simulink model "TADPOLEValveControl"  (R2024b)
settings: Solver=VariableStepAuto  StartTime=0.0  StopTime=100  RelTol=1e-3
values from neighbouring files (symbols this model uses):
  actuator_delay = 0.1131    [TADPOLEControl.m]
  ipaDensityArray = 0.02836    [ipaangle2mdot.m]
  ipaPressureArray = 0.638    [ipaangle2mdot.m]
  oxDensityArray = fuelData(1,:)    [MDotODE.m]    (also in oxangle2mdot.m)
  oxPressureArray = fuelData(2,:)    [MDotODE.m]    (also in oxangle2mdot.m)
undefined symbols (not defined in the file or in its folder): consts, DiscIntNeverNeededParam, Ki1, KiIPA, KiOX, Kp1, KpIPA, KpOX, model_error, simData, thrustArray
libraries: dspobslib x5, dspsrcs4 x2
settings Model: Creator=pplat  LastModifiedBy=pplat
settings DebuggingCC: AlgebraicLoopMsg=none

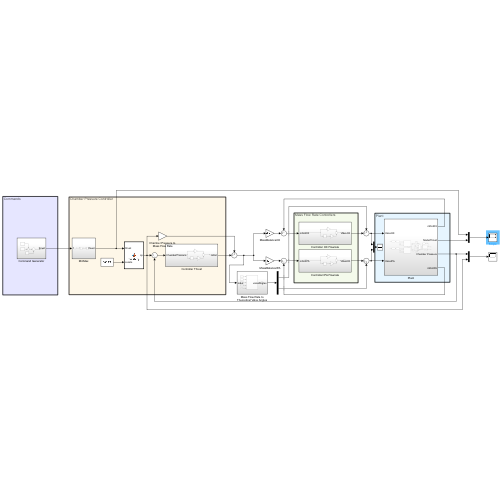
[thumbnail: Simulink's stored preview of the top-level diagram]
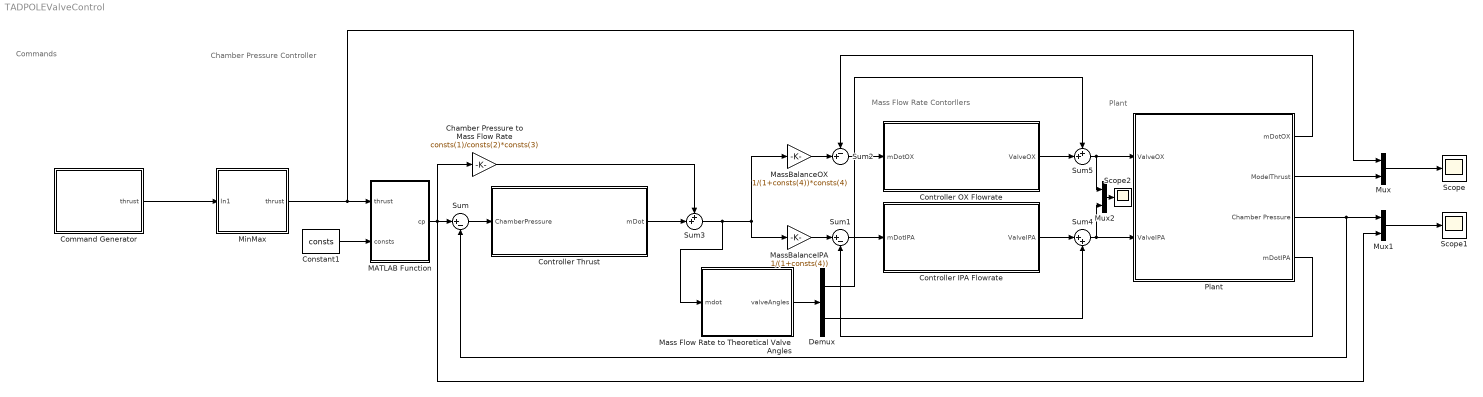
== system TADPOLEValveControl ==
  note: Plant
  note: Mass Flow Rate Contorllers
  note: Chamber Pressure Controller
  note: Commands
  Chamber Pressure to Mass Flow Rate : Gain  Gain=consts(1)/consts(2)*consts(3)
  Command Generator : Subsystem
  Constant1 : Constant  Value=consts
  Controller IPA Flowrate : Subsystem
  Controller OX Flowrate : Subsystem
  Controller Thrust : Subsystem
  Demux : Demux  Outputs=2
  MATLAB Function : MATLAB Function  TreatAsAtomicUnit=on
  "Mass Flow Rate to Theoretical Valve Angles " : Subsystem
  MassBalanceIPA : Gain  Gain=1/(1+consts(4))
  MassBalanceOX : Gain  Gain=1/(1+consts(4))*consts(4)
  MinMax : Subsystem
  Mux : Mux  Inputs=2
  Mux1 : Mux  Inputs=2
  Mux2 : Mux  Inputs=2
  Plant : Subsystem
  Scope : Scope
  Scope1 : Scope
  Scope2 : Scope
  Sum : Sum  Inputs=|+-
  Sum1 : Sum  Inputs=|+-
  Sum2 : Sum  Inputs=-+|
  Sum3 : Sum  Inputs=++|
  Sum4 : Sum  Inputs=|++
  Sum5 : Sum  Inputs=++|
  wires:
  Constant1/1 -> MATLAB Function/2(consts)
  Command Generator/1(thrust) -> MinMax/1(In1)
  Plant/2(ModelThrust) -> Mux/2
  MinMax/1(thrust) -> MATLAB Function/1(thrust), Mux/1
  Mux/1 -> Scope/1
  Sum/1 -> Controller Thrust/1(ChamberPressure)
  Sum1/1 -> Controller IPA Flowrate/1(mDotIPA)
  MassBalanceOX/1 -> Sum2/2
  Sum2/1 -> Controller OX Flowrate/1(mDotOX)
  Plant/1(mDotOX) -> Sum2/1
  Plant/4(mDotIPA) -> Sum1/2
  Plant/3(Chamber Pressure) -> Sum/2, Mux1/1
  Mux1/1 -> Scope1/1
  MATLAB Function/1(cp) -> Chamber Pressure to Mass Flow Rate/1, Mux1/2, Sum/1
  Controller Thrust/1(mDot) -> Sum3/2
  Chamber Pressure to Mass Flow Rate/1 -> Sum3/1
  Sum3/1 -> "Mass Flow Rate to Theoretical Valve Angles "/1(mdot), MassBalanceIPA/1, MassBalanceOX/1
  MassBalanceIPA/1 -> Sum1/1
  Controller IPA Flowrate/1(ValveIPA) -> Sum4/1
  Sum4/1 -> Mux2/2, Plant/2(ValveIPA)
  Controller OX Flowrate/1(ValveOX) -> Sum5/2
  Sum5/1 -> Mux2/1, Plant/1(ValveOX)
  "Mass Flow Rate to Theoretical Valve Angles "/1(valveAngles) -> Demux/1
  Demux/1 -> Sum5/1
  Demux/2 -> Sum4/2
  Mux2/1 -> Scope2/1

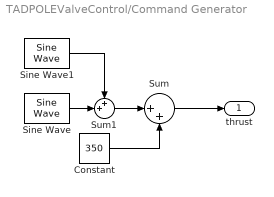
== system TADPOLEValveControl/Command Generator ==
  Constant : Constant  Value=350
  Sine Wave : dspsrcs4/Sine Wave  Amplitude=75  Frequency=0.05  Phase=0  SampleMode=Discrete  OutComplex=Real  CompMethod=Trigonometric fcn  TableSize=Speed  SampleTime=1/60  SamplesPerFrame=1  ResetState=Restart at time zero  OutputFrames=off  dataType=double  wordLen=16  udDataType=sfix(16)  fracBitsMode=Best precision  numFracBits=15  OutDataTypeStr=double  LastOutDataTypeStr=double
  Sine Wave1 : dspsrcs4/Sine Wave  Amplitude=40  Frequency=0.21  Phase=0  SampleMode=Discrete  OutComplex=Real  CompMethod=Trigonometric fcn  TableSize=Speed  SampleTime=1/60  SamplesPerFrame=1  ResetState=Restart at time zero  OutputFrames=off  dataType=double  wordLen=16  udDataType=sfix(16)  fracBitsMode=Best precision  numFracBits=15  OutDataTypeStr=double  LastOutDataTypeStr=double
  Sum : Sum  Inputs=|++
  Sum1 : Sum  Inputs=++|
  thrust : Outport
  wires:
  Sum/1 -> thrust/1
  Constant/1 -> Sum/2
  Sine Wave/1 -> Sum1/2
  Sum1/1 -> Sum/1
  Sine Wave1/1 -> Sum1/1

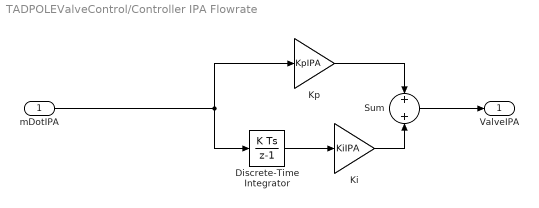
== system TADPOLEValveControl/Controller IPA Flowrate ==
  mDotIPA : Inport
  Discrete-Time Integrator : DiscreteIntegrator  SampleTime=-1  ICPrevOutput=DiscIntNeverNeededParam  ICPrevScaledInput=DiscIntNeverNeededParam
  Ki : Gain  Gain=KiIPA
  Kp : Gain  Gain=KpIPA
  Sum : Sum  Inputs=+|+
  ValveIPA : Outport
  wires:
  mDotIPA/1 -> Discrete-Time Integrator/1, Kp/1
  Kp/1 -> Sum/1
  Ki/1 -> Sum/2
  Sum/1 -> ValveIPA/1
  Discrete-Time Integrator/1 -> Ki/1

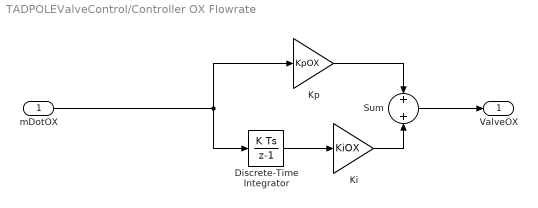
== system TADPOLEValveControl/Controller OX Flowrate ==
  mDotOX : Inport
  Discrete-Time Integrator : DiscreteIntegrator  SampleTime=-1  ICPrevOutput=DiscIntNeverNeededParam  ICPrevScaledInput=DiscIntNeverNeededParam
  Ki : Gain  Gain=KiOX
  Kp : Gain  Gain=KpOX
  Sum : Sum  Inputs=+|+
  ValveOX : Outport
  wires:
  mDotOX/1 -> Discrete-Time Integrator/1, Kp/1
  Kp/1 -> Sum/1
  Ki/1 -> Sum/2
  Sum/1 -> ValveOX/1
  Discrete-Time Integrator/1 -> Ki/1

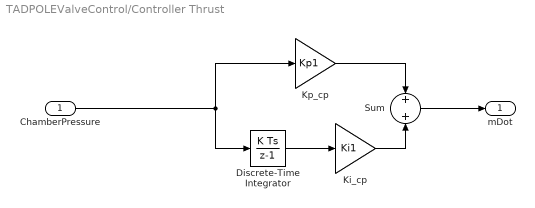
== system TADPOLEValveControl/Controller Thrust ==
  ChamberPressure : Inport
  Discrete-Time Integrator : DiscreteIntegrator  SampleTime=-1  ICPrevOutput=DiscIntNeverNeededParam  ICPrevScaledInput=DiscIntNeverNeededParam
  Ki_cp : Gain  Gain=Ki1
  Kp_cp : Gain  Gain=Kp1
  Sum : Sum  Inputs=+|+
  mDot : Outport
  wires:
  ChamberPressure/1 -> Discrete-Time Integrator/1, Kp_cp/1
  Kp_cp/1 -> Sum/1
  Ki_cp/1 -> Sum/2
  Sum/1 -> mDot/1
  Discrete-Time Integrator/1 -> Ki_cp/1

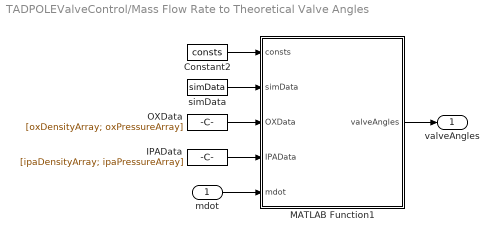
== system TADPOLEValveControl/Mass Flow Rate to Theoretical Valve Angles  ==
  mdot : Inport
  Constant2 : Constant  Value=consts
  IPAData : Constant  Value=[ipaDensityArray; ipaPressureArray]
  MATLAB Function1 : MATLAB Function  TreatAsAtomicUnit=on
  OXData : Constant  Value=[oxDensityArray; oxPressureArray]
  simData : Constant  Value=simData
  valveAngles : Outport
  wires:
  Constant2/1 -> MATLAB Function1/1(consts)
  simData/1 -> MATLAB Function1/2(simData)
  IPAData/1 -> MATLAB Function1/4(IPAData)
  OXData/1 -> MATLAB Function1/3(OXData)
  mdot/1 -> MATLAB Function1/5(mdot)
  MATLAB Function1/1(valveAngles) -> valveAngles/1

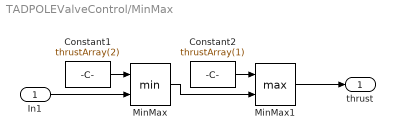
== system TADPOLEValveControl/MinMax ==
  In1 : Inport
  Constant1 : Constant  Value=thrustArray(2)
  Constant2 : Constant  Value=thrustArray(1)
  MinMax : MinMax  Inputs=2
  MinMax1 : MinMax  Function=max  Inputs=2
  thrust : Outport
  wires:
  Constant2/1 -> MinMax1/1
  Constant1/1 -> MinMax/1
  MinMax/1 -> MinMax1/2
  In1/1 -> MinMax/2
  MinMax1/1 -> thrust/1

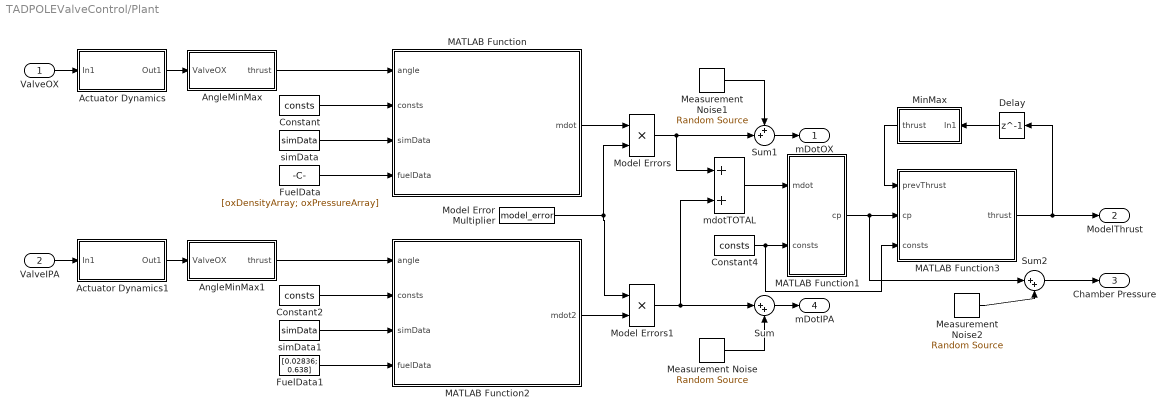
== system TADPOLEValveControl/Plant ==
  ValveOX : Inport
  ValveIPA : Inport  Port=2
  Actuator Dynamics : Subsystem
  Actuator Dynamics1 : Subsystem
  AngleMinMax : Subsystem
  AngleMinMax1 : Subsystem
  Constant : Constant  Value=consts
  Constant2 : Constant  Value=consts
  Constant4 : Constant  Value=consts
  Delay : Delay  DelayLength=1  InitialCondition=0  InputProcessing=Columns as channels (frame based)
  FuelData : Constant  Value=[oxDensityArray; oxPressureArray]
  FuelData1 : Constant  Value=[0.02836; 0.638]
  MATLAB Function : MATLAB Function  TreatAsAtomicUnit=on
  MATLAB Function1 : MATLAB Function  TreatAsAtomicUnit=on
  MATLAB Function2 : MATLAB Function  TreatAsAtomicUnit=on
  MATLAB Function3 : MATLAB Function  TreatAsAtomicUnit=on
  Measurement Noise : dspobslib/Random Source  SrcType=Gaussian  NormMethod=Ziggurat  CltLength=12  MinVal=0  MaxVal=1  MeanVal=0  VarVal=noise_var_outputs  RepMode=Not repeatable  rawSeed=1  IsInherit=off  SampMode=Continuous  SampTime=1  SampFrame=1  DataType=Double  OutComplex=Real  OutputFrames=off
  Measurement Noise1 : dspobslib/Random Source  SrcType=Gaussian  NormMethod=Ziggurat  CltLength=12  MinVal=0  MaxVal=1  MeanVal=0  VarVal=noise_var_outputs  RepMode=Not repeatable  rawSeed=1  IsInherit=off  SampMode=Continuous  SampTime=1  SampFrame=1  DataType=Double  OutComplex=Real  OutputFrames=off
  Measurement Noise2 : dspobslib/Random Source  SrcType=Gaussian  NormMethod=Ziggurat  CltLength=12  MinVal=0  MaxVal=1  MeanVal=0  VarVal=noise_var_outputs  RepMode=Not repeatable  rawSeed=1  IsInherit=off  SampMode=Continuous  SampTime=1  SampFrame=1  DataType=Double  OutComplex=Real  OutputFrames=off
  MinMax : Subsystem
  Model Error Multiplier : Constant  Value=model_error
  Model Errors : Product
  Model Errors1 : Product
  Sum : Sum  Inputs=|++
  Sum1 : Sum  Inputs=++|
  Sum2 : Sum  Inputs=|++
  mdotTOTAL : Sum
  simData : Constant  Value=simData
  simData1 : Constant  Value=simData
  mDotOX : Outport
  ModelThrust : Outport  Port=2
  Chamber Pressure : Outport  Port=3
  mDotIPA : Outport  Port=4
  wires:
  Constant/1 -> MATLAB Function/2(consts)
  FuelData/1 -> MATLAB Function/4(fuelData)
  FuelData1/1 -> MATLAB Function2/4(fuelData)
  Constant2/1 -> MATLAB Function2/2(consts)
  Constant4/1 -> MATLAB Function3/3(consts), MATLAB Function1/2(consts)
  mdotTOTAL/1 -> MATLAB Function1/1(mdot)
  Delay/1 -> MinMax/1(In1)
  MinMax/1(thrust) -> MATLAB Function3/1(prevThrust)
  simData/1 -> MATLAB Function/3(simData)
  simData1/1 -> MATLAB Function2/3(simData)
  MATLAB Function3/1(thrust) -> ModelThrust/1, Delay/1
  MATLAB Function1/1(cp) -> Sum2/1, MATLAB Function3/2(cp)
  ValveOX/1 -> Actuator Dynamics/1(In1)
  Actuator Dynamics/1(Out1) -> AngleMinMax/1(ValveOX)
  ValveIPA/1 -> Actuator Dynamics1/1(In1)
  Actuator Dynamics1/1(Out1) -> AngleMinMax1/1(ValveOX)
  Sum/1 -> mDotIPA/1
  Measurement Noise/1 -> Sum/2
  Sum1/1 -> mDotOX/1
  Measurement Noise1/1 -> Sum1/1
  Measurement Noise2/1 -> Sum2/2
  Sum2/1 -> Chamber Pressure/1
  Model Errors/1 -> Sum1/2, mdotTOTAL/1
  MATLAB Function/1(mdot) -> Model Errors/1
  MATLAB Function2/1(mdot2) -> Model Errors1/2
  Model Errors1/1 -> mdotTOTAL/2, Sum/1
  Model Error Multiplier/1 -> Model Errors1/1, Model Errors/2
  AngleMinMax/1(thrust) -> MATLAB Function/1(angle)
  AngleMinMax1/1(thrust) -> MATLAB Function2/1(angle)

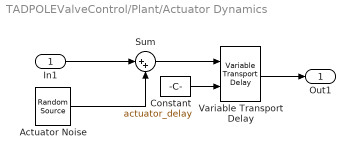
== system TADPOLEValveControl/Plant/Actuator Dynamics ==
  In1 : Inport
  Actuator Noise : dspobslib/Random Source  SrcType=Gaussian  NormMethod=Ziggurat  CltLength=12  MinVal=0  MaxVal=1  MeanVal=0  VarVal=noise_var_actuators  RepMode=Not repeatable  rawSeed=1  IsInherit=off  SampMode=Continuous  SampTime=1  SampFrame=1  DataType=Double  OutComplex=Real  OutputFrames=off
  Constant : Constant  Value=actuator_delay
  Sum : Sum  Inputs=|++
  Variable Transport Delay : VariableTransportDelay  VariableDelayType=Variable transport delay  MaximumDelay=10  MaximumPoints=2048
  Out1 : Outport
  wires:
  Actuator Noise/1 -> Sum/2
  In1/1 -> Sum/1
  Constant/1 -> Variable Transport Delay/2
  Variable Transport Delay/1 -> Out1/1
  Sum/1 -> Variable Transport Delay/1

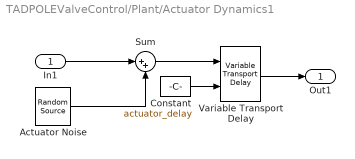
== system TADPOLEValveControl/Plant/Actuator Dynamics1 ==
  In1 : Inport
  Actuator Noise : dspobslib/Random Source  SrcType=Gaussian  NormMethod=Ziggurat  CltLength=12  MinVal=0  MaxVal=1  MeanVal=0  VarVal=noise_var_actuators  RepMode=Not repeatable  rawSeed=1  IsInherit=off  SampMode=Continuous  SampTime=1  SampFrame=1  DataType=Double  OutComplex=Real  OutputFrames=off
  Constant : Constant  Value=actuator_delay
  Sum : Sum  Inputs=|++
  Variable Transport Delay : VariableTransportDelay  VariableDelayType=Variable transport delay  MaximumDelay=10  MaximumPoints=2048
  Out1 : Outport
  wires:
  Actuator Noise/1 -> Sum/2
  In1/1 -> Sum/1
  Constant/1 -> Variable Transport Delay/2
  Variable Transport Delay/1 -> Out1/1
  Sum/1 -> Variable Transport Delay/1

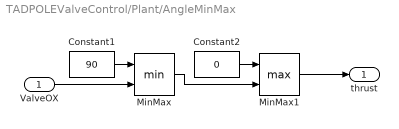
== system TADPOLEValveControl/Plant/AngleMinMax ==
  ValveOX : Inport
  Constant1 : Constant  Value=90
  Constant2 : Constant  Value=0
  MinMax : MinMax  Inputs=2
  MinMax1 : MinMax  Function=max  Inputs=2
  thrust : Outport
  wires:
  Constant2/1 -> MinMax1/1
  Constant1/1 -> MinMax/1
  MinMax/1 -> MinMax1/2
  ValveOX/1 -> MinMax/2
  MinMax1/1 -> thrust/1

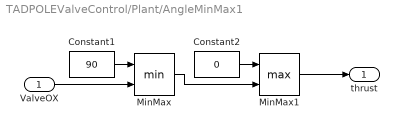
== system TADPOLEValveControl/Plant/AngleMinMax1 ==
  ValveOX : Inport
  Constant1 : Constant  Value=90
  Constant2 : Constant  Value=0
  MinMax : MinMax  Inputs=2
  MinMax1 : MinMax  Function=max  Inputs=2
  thrust : Outport
  wires:
  Constant2/1 -> MinMax1/1
  Constant1/1 -> MinMax/1
  MinMax/1 -> MinMax1/2
  ValveOX/1 -> MinMax/2
  MinMax1/1 -> thrust/1

== system TADPOLEValveControl/Plant/MinMax ==
  In1 : Inport
  Constant1 : Constant  Value=thrustArray(2)
  Constant2 : Constant  Value=thrustArray(1)
  MinMax : MinMax  Inputs=2
  MinMax1 : MinMax  Function=max  Inputs=2
  thrust : Outport
  wires:
  Constant2/1 -> MinMax1/1
  Constant1/1 -> MinMax/1
  MinMax/1 -> MinMax1/2
  In1/1 -> MinMax/2
  MinMax1/1 -> thrust/1

== matlab function TADPOLEValveControl/Plant/MATLAB Function ==
  data: angle input; mdot output; consts input; simData input; fuelData input
function mdot = oxangle2mdot(angle, consts, simData, fuelData)

    % Conversion Factors and LookUp Arrays
    conversionFactors = [0.004329 60 0.000453592 61023.7];
    subCritVArray = [0.000, 0.070, 0.161, 0.378, 0.670, 1.000, 1.450, 2.050, 2.780, 3.710, 4.960];
    valveAngleArray = [0, 9, 18, 27, 36, 45, 54, 63, 72, 81, 90];
    tempArray = [55, 60, 65, 70, 75, 80, 85, 90, 95, 100, 105, 110, ...
    115, 120, 125, 130, 135, 140, 145, 150];
    oxDensityArray = fuelData(1,:);
    oxPressureArray = fuelData(2,:);

    % cV lookup based off of angle
    subCritV = interp1(valveAngleArray, subCritVArray, angle);

    % ox
    throat = 0.00989;
    cd = 0.975;

    % density and vapour pressure ox
    simData(4);
    density_cv = interp1(tempArray, oxDensityArray, simData(4));
    p_vap = interp1(tempArray, oxPressureArray, simData(4));
    density_valve = interp1(tempArray, oxDensityArray, simData(3));

    %Generates mdot
    alpha = conversionFactors(1)*conversionFactors(2);
    gamma = cd^2*throat^2*2*density_cv*(consts(3)*12);
    beta = conversionFactors(3)*conversionFactors(4);
    deltaP = simData(1)-p_vap;
    mdot = sqrt(subCritV^2*density_valve*(deltaP)*gamma /...
        (alpha^2*gamma*beta + subCritV^2*density_valve));
end

== matlab function TADPOLEValveControl/MATLAB Function ==
  data: thrust input; cp output; consts input
function cp = thrust2cp(thrust, consts)
  
    thrustArray = [220, 550];
    c_fArray = [1.12, 1.3];
    c_f = interp1(thrustArray, c_fArray, thrust);
    cp = thrust / (c_f*consts(1));
end

== matlab function TADPOLEValveControl/Plant/MATLAB Function1 ==
  data: mdot input; cp output; consts input
function cp = mdot2cp(mdot, consts)
    
    cp = mdot*consts(2) / (consts(1)*consts(3));
end

== matlab function TADPOLEValveControl/Plant/MATLAB Function2 ==
  data: angle input; mdot2 output; consts input; simData input; fuelData input
function mdot2 = ipaangle2mdot(angle, consts, simData, fuelData)

    % Conversion Factors and LookUp Arrays
    conversionFactors = [0.004329 60 0.000453592 61023.7];
    subCritVArray = [0.000, 0.070, 0.161, 0.378, 0.670, 1.000, 1.450, 2.050, 2.780, 3.710, 4.960];
    valveAngleArray = [0, 9, 18, 27, 36, 45, 54, 63, 72, 81, 90];
    tempArray = [55, 60, 65, 70, 75, 80, 85, 90, 95, 100, 105, 110, ...
    115, 120, 125, 130, 135, 140, 145, 150];
    ipaDensityArray = fuelData(1,:);
    ipaPressureArray = fuelData(2,:);

    % cV lookup based off of angle
    subCritV = interp1(valveAngleArray, subCritVArray, angle);

    % ox
    throat = 0.00989;
    cd = 0.975;

    % density and vapour pressure ox
    simData(4);
    density_cv = ipaDensityArray;
    p_vap = ipaPressureArray;
    density_valve = ipaDensityArray;

    %Generates mdot
    alpha = conversionFactors(1)*conversionFactors(2);
    gamma = cd^2*throat^2*2*density_cv*(consts(3)*12);
    beta = conversionFactors(3)*conversionFactors(4);
    deltaP = simData(1)-p_vap;
    mdot2 = sqrt(subCritV^2*density_valve*(deltaP)*gamma /...
        (alpha^2*gamma*beta + subCritV^2*density_valve));
end

== matlab function TADPOLEValveControl/Plant/MATLAB Function3 ==
  data: prevThrust input; cp input; thrust output; consts input
function thrust = cp2thrust(prevThrust, cp, consts)
  
    thrustArray = [220, 550];
    c_fArray = [1.12, 1.3];
    c_f = interp1(thrustArray, c_fArray, prevThrust);
    thrust = cp*c_f*consts(1);
end

== matlab function TADPOLEValveControl/Mass Flow Rate to Theoretical Valve Angles /MATLAB Function1 ==
  data: consts input; simData input; OXData input; IPAData input; mdot input; valveAngles output
function valveAngles = mdot2valves(consts, simData, OXData, IPAData, mdot)
   
    % Conversion Factors and LookUp Arrays
    conversionFactors = [0.004329 60 0.000453592 61023.7];
    subCritVArray = [0.000, 0.070, 0.161, 0.378, 0.670, 1.000, 1.450, 2.050, 2.780, 3.710, 4.960];
    valveAngleArray = [0, 9, 18, 27, 36, 45, 54, 63, 72, 81, 90];
    tempArray = [55, 60, 65, 70, 75, 80, 85, 90, 95, 100, 105, 110, ...
    115, 120, 125, 130, 135, 140, 145, 150];
    oxDensityArray = OXData(1,:);
    oxPressureArray = OXData(2,:);

    % Mass balance
    mdot_OX = mdot / (1+consts(4))*consts(4);
    mdot_IPA = mdot / (1+consts(4));

    % ox/ipa 
    throat = 0.00989;
    cd = 0.975;
    densityOX_cv = interp1(tempArray, oxDensityArray, simData(4));
    densityIPA_cv = IPAData(1);
    densityOX_valve = interp1(tempArray, oxDensityArray, simData(3));
    densityIPA_valve = IPAData(1);
    P_vap_OX = interp1(tempArray, oxPressureArray, simData(4));
    P_vap_IPA = IPAData(2);

    % Cavitating venturis
    P_in_OX = (mdot_OX / (cd*throat))^2 / (2*densityOX_cv*(consts(3)*12))...
        + P_vap_OX;
    P_in_IPA = (mdot_IPA / (cd*throat))^2 / (2*densityIPA_cv*(consts(3)*12))...
        + P_vap_IPA;

    % DeltaPs
    deltaP_OX = max(0.0001, (simData(1)-P_in_OX));
    deltaP_IPA = max(0.0001, (simData(2)-P_in_IPA));

    % Sub Critical Venturis
    subCritV_OX = mdot_OX*conversionFactors(1)*conversionFactors(2)*...
        sqrt(conversionFactors(3)*conversionFactors(4) /...
        (deltaP_OX*densityOX_valve));
    subCritV_IPA = mdot_IPA*conversionFactors(1)*conversionFactors(2)*...
        sqrt(conversionFactors(3)*conversionFactors(4) /...
        (deltaP_IPA*densityIPA_valve));

    valveOX = interp1(subCritVArray, valveAngleArray, subCritV_OX);
    valveIPA = interp1(subCritVArray, valveAngleArray, subCritV_IPA);

    valveAngles = [valveOX, valveIPA];
end
